simulink model "Inverter_Simulink_Simutation"  (R2019a)
settings: Solver=VariableStepAuto  StartTime=0.0  StopTime=.01  FixedStep=1e-9  RelTol=1e-3
libraries: powerlib x12, powerlib_meascontrol x2
settings Model: Creator=Olive  LastModifiedBy=oliverrodriguez
settings DataIOCC: ReturnWorkspaceOutputs=off
settings DebuggingCC: PregeneratedLibrarySubsystemCodeDiagnostic=none  ArithmeticOperatorsInVariantConditions=warning
settings SFSimCC: SimUseLocalCustomCode=off
settings RTWCC: RTWUseLocalCustomCode=off

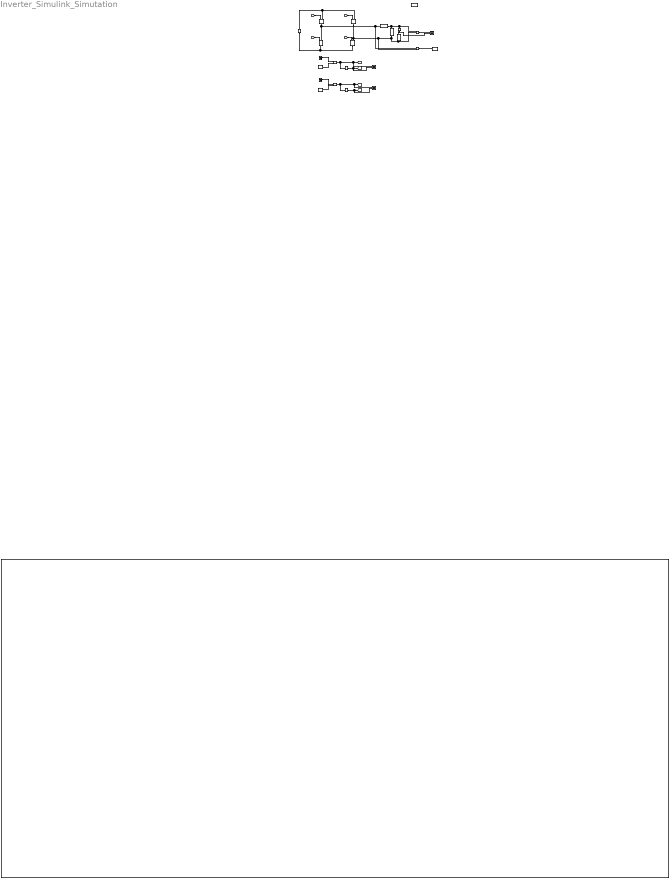
== system Inverter_Simulink_Simutation ==
  Current Measurement : powerlib/Measurements/Current Measurement  PhasorSimulation=off  OutputType=Complex  PSBequivalent=0
      settings: SourceProductName=Simscape Electrical
  DC Voltage Source : powerlib/Electrical Sources/DC Voltage Source  Amplitude=1  Measurements=None
      settings: SourceProductName=Simscape Electrical
  Dashboard Scope : DashboardScope
  GreaterThanOrEqual : RelationalOperator  OutDataTypeStr=boolean  RndMeth=Simplest
  GreaterThanOrEqual1 : RelationalOperator  OutDataTypeStr=boolean  RndMeth=Simplest
  Logical Operator : Logic  Operator=NOT  AllPortsSameDT=off  OutDataTypeStr=boolean
  Logical Operator1 : Logic  Operator=NOT  AllPortsSameDT=off  OutDataTypeStr=boolean
  Mosfet{,1..3} (4 alike) : powerlib/Power Electronics/Mosfet  Ron=0.001  Lon=0  Rd=0.01  Vfd=0  IC=0  Rs=1e5  Cs=inf  Measurements=off
      settings: SourceProductName=Simscape Electrical
  Scope : Scope  NumInputPorts=2
  Scope1 : Scope  NumInputPorts=2
  Scope2 : Scope  NumInputPorts=2
  Series RLC Branch1 : powerlib/Elements/Series RLC Branch  LConnTagsString=__new0  RConnTagsString=__new0  BranchType=R  Resistance=100000  Inductance=1e-3  SetiL0=off  InitialCurrent=0  Capacitance=1e-6  Setx0=off  InitialVoltage=0  Measurements=None
      settings: SourceProductName=Simscape Electrical
  Series RLC Branch2 : powerlib/Elements/Series RLC Branch  LConnTagsString=__new0  RConnTagsString=__new0  BranchType=C  Resistance=1.7  Inductance=1e-3  SetiL0=off  InitialCurrent=0  Capacitance=168e-6  Setx0=off  InitialVoltage=0  Measurements=None
      settings: SourceProductName=Simscape Electrical
  Series RLC Branch3 : powerlib/Elements/Series RLC Branch  LConnTagsString=__new0  RConnTagsString=__new0  BranchType=L  Resistance=1.7  Inductance=1e-3  SetiL0=off  InitialCurrent=0  Capacitance=1e-6  Setx0=off  InitialVoltage=0  Measurements=None
      settings: SourceProductName=Simscape Electrical
  Sine Wave : Sin  Amplitude=1.0  Frequency=100.*pi  SampleTime=0
  Sine Wave2 : Sin  Amplitude=-1.0  Frequency=100*pi  SampleTime=0
  To Workspace : ToWorkspace  VariableName=SPWM  SampleTime=1e-6
  Triangle Generator : powerlib_meascontrol/Pulse & Signal Generators/Triangle Generator  Freq=4000  Phase=0  Ts=0
      settings: SourceProductName=Simscape Electrical
  Triangle Generator1 : powerlib_meascontrol/Pulse & Signal Generators/Triangle Generator  Freq=4000  Phase=0  Ts=0
      settings: SourceProductName=Simscape Electrical
  Voltage Measurement : powerlib/Measurements/Voltage Measurement  PhasorSimulation=off  OutputType=Complex  PSBequivalent=0
      settings: SourceProductName=Simscape Electrical
  Voltage Measurement1 : powerlib/Measurements/Voltage Measurement  PhasorSimulation=off  OutputType=Complex  PSBequivalent=0
      settings: SourceProductName=Simscape Electrical
  powergui : powerlib/powergui  Priority=1  SimulationMode=Continuous  SampleTime=50e-6  frequency=60  Iterations=50  frequencyindice=0  Pbase=100e6  ErrMax=1e-4  UnitsV=kV  UnitsW=MW  buscounter=0  FunctionMessages=off  echomessages=off  EnableUseOfTLC=off  CurrentSourceSwitches=off  DisableSnubberDevices=off  DisableRonSwitches=off  DisableVfSwitches=off  DisplayEquations=off  AutomaticDiscreteSolvers=off  SolverType=Tustin/Backward Euler (TBE)  Interpol=off  ExternalGateDelay=off  methode=off  Ts=100  x0status=blocks  SPID=on  SwTol=0  HookPort=off  NonlinearTolerance=0  nMaxIteration=15  ContinueOnMaxIteration=off  RestoreLinks=warning  ResistiveCurrentMeasurement=off  Frange=[0:2:500]  Ylog=off  Xlog=on  ShowGrid=off  save=off  variable=ZData  structure=0  ZoomFFT=off  StartTime=0.0  cycles=1  DisplayStyle=1  fundamental=60  FreqAxis=off  MaxFrequency=1000  frequencyindicesteady=1  RmsSteady=1  display=off
      settings: SourceProductName=Simscape Electrical
  wires:
  Sine Wave/1 -> GreaterThanOrEqual/1
  Triangle Generator/1 -> GreaterThanOrEqual/2
  GreaterThanOrEqual/1 -> Scope/1, [A1], Logical Operator/1
  Logical Operator/1 -> Scope/2, [A2]
  Logical Operator1/1 -> Scope1/2, [B2]
  Sine Wave2/1 -> GreaterThanOrEqual1/1
  Triangle Generator1/1 -> GreaterThanOrEqual1/2
  [B1] -> Mosfet3/1
  [A1] -> Mosfet/1
  [A2] -> Mosfet2/1
  [B2] -> Mosfet1/1
  Voltage Measurement1/1 -> To Workspace/1
  Voltage Measurement/1 -> Scope2/1
  Current Measurement/1 -> Scope2/2
  GreaterThanOrEqual1/1 -> Scope1/1, [B1], Logical Operator1/1
  connections:
  Series RLC Branch2/LConn1 -- Voltage Measurement/LConn1 -- Current Measurement/LConn1 -- Series RLC Branch3/LConn1
  DC Voltage Source/RConn1 -- Mosfet3/LConn1 -- Mosfet/LConn1
  DC Voltage Source/LConn1 -- Mosfet1/RConn1 -- Mosfet2/RConn1
  Mosfet3/RConn1 -- Voltage Measurement1/LConn2 -- Series RLC Branch2/RConn1 -- Series RLC Branch1/RConn1 -- Voltage Measurement/LConn2 -- Mosfet1/LConn1
  Mosfet/RConn1 -- Mosfet2/LConn1 -- Voltage Measurement1/LConn1 -- Series RLC Branch3/RConn1
  Current Measurement/RConn1 -- Series RLC Branch1/LConn1
